simulink model "DvrSimKeybdGD_cs"  (R2016a)
settings: Solver=ode5  SolverMode=SingleTasking  StartTime=0.0  StopTime=inf  FixedStep=1/1000  RelTol=1e-3
PreLoadFcn:
  | mbxruntime.callbacks.PreLoadFcn(bdroot);
PostLoadFcn:
  | mbxruntime.callbacks.PostLoadFcn(bdroot);
InitFcn:
  | mbxruntime.callbacks.InitFcn(bdroot);
StartFcn:
  | mbxruntime.callbacks.StartFcn(bdroot);
StopFcn:
  | mbxruntime.callbacks.StopFcn(bdroot);
model workspace (MAT data in the model file):
  mbox_table : struct (value not decoded)
  model_closed = 0
  sim_status = 0
undefined symbols (not defined in the file or in its folder): BMotor1, BMotor2, BrkDelayTime, DControlB, Delay1, Delay2, DiscIntNeverNeededParam, IControlB, JMotor1, JMotor2, PControlB, PreScanCarSimLoadFcn, ratioGearF, ratioGearR, TorqDelayTime, Tstep
undefined symbols (not defined in the file): SteeringColumn, SteeringWheel, WheelL0, WheelL1, WheelR0, WheelR1
libraries: PreScanSimulinkLibrary x35, simulink_extras x26, simulink x26, MyLib x3, Solver_SF x2, pil_lib x1, PreScanUsefulBlocks x1
(part 12 of 12)

== system DvrSimKeybdGD_cs/Audi_A8_Sedan_1/Trajectories/ElapsedTrack1/MuxState/Substitute 90 & 270 deg (and its plurals)/Angle 0-360 deg limiter ==
  Angle [deg] : Inport
  Gain : Gain  Gain=1/360
  Gain1 : Gain  Gain=360
  Rounding Function : Rounding
  Sum : Sum  Inputs=|-+
  LimAngle [deg] : Outport
  wires:
  Gain/1 -> Rounding Function/1
  Rounding Function/1 -> Gain1/1
  Gain1/1 -> Sum/1
  Angle [deg]/1 -> Gain/1, Sum/2
  Sum/1 -> LimAngle [deg]/1

== system DvrSimKeybdGD_cs/Audi_A8_Sedan_1/Trajectories/Traj2State1/Traj2State2/Traj2MuxState_Ext/demux ==
  traj : Inport
  Demux : Demux  Outputs=18
  x : Outport
  y : Outport  Port=2
  z : Outport  Port=3
  velx : Outport  Port=4
  vely : Outport  Port=5
  velz : Outport  Port=6
  R : Outport  Port=7
  P : Outport  Port=8
  Y : Outport  Port=9
  velR : Outport  Port=10
  velP : Outport  Port=11
  velY : Outport  Port=12
  accx : Outport  Port=13
  accy : Outport  Port=14
  accz : Outport  Port=15
  accR : Outport  Port=16
  accP : Outport  Port=17
  accY : Outport  Port=18
  wires:
  Demux/18 -> accY/1
  Demux/17 -> accP/1
  Demux/16 -> accR/1
  Demux/15 -> accz/1
  Demux/14 -> accy/1
  Demux/13 -> accx/1
  Demux/12 -> velY/1
  Demux/11 -> velP/1
  Demux/10 -> velR/1
  Demux/9 -> velz/1
  Demux/8 -> vely/1
  Demux/7 -> velx/1
  Demux/6 -> Y/1
  Demux/5 -> P/1
  traj/1 -> Demux/1
  Demux/4 -> R/1
  Demux/3 -> z/1
  Demux/2 -> y/1
  Demux/1 -> x/1

== system DvrSimKeybdGD_cs/BMW_X5_SUV_1/Trajectories/ElapsedTrack1/MuxState/Substitute 90 & 270 deg (and its plurals)/Angle 0-360 deg limiter ==
  Angle [deg] : Inport
  Gain : Gain  Gain=1/360
  Gain1 : Gain  Gain=360
  Rounding Function : Rounding
  Sum : Sum  Inputs=|-+
  LimAngle [deg] : Outport
  wires:
  Gain/1 -> Rounding Function/1
  Rounding Function/1 -> Gain1/1
  Gain1/1 -> Sum/1
  Angle [deg]/1 -> Gain/1, Sum/2
  Sum/1 -> LimAngle [deg]/1

== system DvrSimKeybdGD_cs/BMW_X5_SUV_1/Trajectories/Traj2State1/Traj2State2/Traj2MuxState_Ext/demux ==
  traj : Inport
  Demux : Demux  Outputs=18
  x : Outport
  y : Outport  Port=2
  z : Outport  Port=3
  velx : Outport  Port=4
  vely : Outport  Port=5
  velz : Outport  Port=6
  R : Outport  Port=7
  P : Outport  Port=8
  Y : Outport  Port=9
  velR : Outport  Port=10
  velP : Outport  Port=11
  velY : Outport  Port=12
  accx : Outport  Port=13
  accy : Outport  Port=14
  accz : Outport  Port=15
  accR : Outport  Port=16
  accP : Outport  Port=17
  accY : Outport  Port=18
  wires:
  Demux/18 -> accY/1
  Demux/17 -> accP/1
  Demux/16 -> accR/1
  Demux/15 -> accz/1
  Demux/14 -> accy/1
  Demux/13 -> accx/1
  Demux/12 -> velY/1
  Demux/11 -> velP/1
  Demux/10 -> velR/1
  Demux/9 -> velz/1
  Demux/8 -> vely/1
  Demux/7 -> velx/1
  Demux/6 -> Y/1
  Demux/5 -> P/1
  traj/1 -> Demux/1
  Demux/4 -> R/1
  Demux/3 -> z/1
  Demux/2 -> y/1
  Demux/1 -> x/1

== system DvrSimKeybdGD_cs/BMW_Z3_Convertible_1/Trajectories/ElapsedTrack1/MuxState/Substitute 90 & 270 deg (and its plurals)/Angle 0-360 deg limiter ==
  Angle [deg] : Inport
  Gain : Gain  Gain=1/360
  Gain1 : Gain  Gain=360
  Rounding Function : Rounding
  Sum : Sum  Inputs=|-+
  LimAngle [deg] : Outport
  wires:
  Gain/1 -> Rounding Function/1
  Rounding Function/1 -> Gain1/1
  Gain1/1 -> Sum/1
  Angle [deg]/1 -> Gain/1, Sum/2
  Sum/1 -> LimAngle [deg]/1

== system DvrSimKeybdGD_cs/BMW_Z3_Convertible_1/Trajectories/Traj2State1/Traj2State2/Traj2MuxState_Ext/demux ==
  traj : Inport
  Demux : Demux  Outputs=18
  x : Outport
  y : Outport  Port=2
  z : Outport  Port=3
  velx : Outport  Port=4
  vely : Outport  Port=5
  velz : Outport  Port=6
  R : Outport  Port=7
  P : Outport  Port=8
  Y : Outport  Port=9
  velR : Outport  Port=10
  velP : Outport  Port=11
  velY : Outport  Port=12
  accx : Outport  Port=13
  accy : Outport  Port=14
  accz : Outport  Port=15
  accR : Outport  Port=16
  accP : Outport  Port=17
  accY : Outport  Port=18
  wires:
  Demux/18 -> accY/1
  Demux/17 -> accP/1
  Demux/16 -> accR/1
  Demux/15 -> accz/1
  Demux/14 -> accy/1
  Demux/13 -> accx/1
  Demux/12 -> velY/1
  Demux/11 -> velP/1
  Demux/10 -> velR/1
  Demux/9 -> velz/1
  Demux/8 -> vely/1
  Demux/7 -> velx/1
  Demux/6 -> Y/1
  Demux/5 -> P/1
  traj/1 -> Demux/1
  Demux/4 -> R/1
  Demux/3 -> z/1
  Demux/2 -> y/1
  Demux/1 -> x/1

== system DvrSimKeybdGD_cs/Ford_Fiesta_Hatchback_1/Trajectories/ElapsedTrack1/MuxState/Substitute 90 & 270 deg (and its plurals)/Angle 0-360 deg limiter ==
  Angle [deg] : Inport
  Gain : Gain  Gain=1/360
  Gain1 : Gain  Gain=360
  Rounding Function : Rounding
  Sum : Sum  Inputs=|-+
  LimAngle [deg] : Outport
  wires:
  Gain/1 -> Rounding Function/1
  Rounding Function/1 -> Gain1/1
  Gain1/1 -> Sum/1
  Angle [deg]/1 -> Gain/1, Sum/2
  Sum/1 -> LimAngle [deg]/1

== system DvrSimKeybdGD_cs/Ford_Fiesta_Hatchback_1/Trajectories/Traj2State1/Traj2State2/Traj2MuxState_Ext/demux ==
  traj : Inport
  Demux : Demux  Outputs=18
  x : Outport
  y : Outport  Port=2
  z : Outport  Port=3
  velx : Outport  Port=4
  vely : Outport  Port=5
  velz : Outport  Port=6
  R : Outport  Port=7
  P : Outport  Port=8
  Y : Outport  Port=9
  velR : Outport  Port=10
  velP : Outport  Port=11
  velY : Outport  Port=12
  accx : Outport  Port=13
  accy : Outport  Port=14
  accz : Outport  Port=15
  accR : Outport  Port=16
  accP : Outport  Port=17
  accY : Outport  Port=18
  wires:
  Demux/18 -> accY/1
  Demux/17 -> accP/1
  Demux/16 -> accR/1
  Demux/15 -> accz/1
  Demux/14 -> accy/1
  Demux/13 -> accx/1
  Demux/12 -> velY/1
  Demux/11 -> velP/1
  Demux/10 -> velR/1
  Demux/9 -> velz/1
  Demux/8 -> vely/1
  Demux/7 -> velx/1
  Demux/6 -> Y/1
  Demux/5 -> P/1
  traj/1 -> Demux/1
  Demux/4 -> R/1
  Demux/3 -> z/1
  Demux/2 -> y/1
  Demux/1 -> x/1

== system DvrSimKeybdGD_cs/Roewe_550_S_Sedan_1/CarSim_Vehicle/CarSim2PreScan_BUS/Wheel/Convert CarSim to PreScan Wheel Position/Transformation_WheelGlobal2WheelLocal ==
  SprungMass_Pos_Global[x;y;z][m] : Inport
  SprungMass_Angle_Global[x;y;z][deg] : Inport  Port=2
  Wheels_Pos_Global[x;y;z][m] : Inport  Port=3
  D2R : Gain  Gain=pi/180
  Dot Product : DotProduct  InputSameDT=on  OutDataTypeStr=Inherit: Inherit via internal rule
  Dot Product1 : DotProduct  InputSameDT=on  OutDataTypeStr=Inherit: Inherit via internal rule
  Dot Product2 : DotProduct  InputSameDT=on  OutDataTypeStr=Inherit: Inherit via internal rule
  Fcn10 : Fcn  Expr=cos(u(1))*sin(u(2))*sin(u(3))-sin(u(1))*cos(u(3))
  Fcn11 : Fcn  Expr=cos(u(1))*sin(u(2))*cos(u(3))+sin(u(1))*sin(u(3))
  Fcn12 : Fcn  Expr=sin(u(1))*cos(u(2))
  Fcn13 : Fcn  Expr=sin(u(1))*sin(u(2))*sin(u(3))+cos(u(1))*cos(u(3))
  Fcn14 : Fcn  Expr=sin(u(1))*sin(u(2))*cos(u(3))-cos(u(1))*sin(u(3))
  Fcn15 : Fcn  Expr=-sin(u(2))
  Fcn16 : Fcn  Expr=cos(u(2))*sin(u(3))
  Fcn17 : Fcn  Expr=cos(u(2))*cos(u(3))
  Fcn9 : Fcn  Expr=cos(u(1))*cos(u(2))
  Mux : Mux
  Mux1 : Mux  Inputs=9
  Mux3 : Mux  Inputs=3
  PreScan_WheelShiftFL : Subsystem  mask(Translation node configuration){tp=Rear-Left Wheel}
      mask prompts: tp "Type"
      mask init:
      | x_ini_VRML = 2.701790; 
      | y_ini_VRML = 0.665750; 
      | z_ini_VRML = 0.317714;
      mask TypeOptions tp: Front-Left Wheel | Front-Right Wheel | Rear-Left Wheel | Rear-Right Wheel | Left Seat | Right Seat
  PreScan_WheelShiftFR : Subsystem  mask(Translation node configuration){tp=Rear-Right Wheel}
      mask prompts: tp "Type"
      mask init:
      | x_ini_VRML = 2.701790; 
      | y_ini_VRML = -0.665750; 
      | z_ini_VRML = 0.317714;
      mask TypeOptions tp: Front-Left Wheel | Front-Right Wheel | Rear-Left Wheel | Rear-Right Wheel | Left Seat | Right Seat
  PreScan_WheelShiftRL : Subsystem  mask(Translation node configuration){tp=Front-Left Wheel}
      mask prompts: tp "Type"
      mask init:
      | x_ini_VRML = 0.000000; 
      | y_ini_VRML = 0.665750; 
      | z_ini_VRML = 0.317714;
      mask TypeOptions tp: Front-Left Wheel | Front-Right Wheel | Rear-Left Wheel | Rear-Right Wheel | Left Seat | Right Seat
  PreScan_WheelShiftRR : Subsystem  mask(Translation node configuration){tp=Front-Right Wheel}
      mask prompts: tp "Type"
      mask init:
      | x_ini_VRML = 0.000000; 
      | y_ini_VRML = -0.665750; 
      | z_ini_VRML = 0.317714;
      mask TypeOptions tp: Front-Left Wheel | Front-Right Wheel | Rear-Left Wheel | Rear-Right Wheel | Left Seat | Right Seat
  Selector : Selector  InputPortWidth=9  IndexOptions=Index vector (dialog)  Indices=[1 2 3]  OutputSizes=1
  Selector1 : Selector  InputPortWidth=9  IndexOptions=Index vector (dialog)  Indices=[4 5 6]  OutputSizes=1
  Selector2 : Selector  InputPortWidth=9  IndexOptions=Index vector (dialog)  Indices=[7 8 9]  OutputSizes=1
  Subsystem : Subsystem
  Sum{1..4} (4 alike) : Sum  Inputs=-+
  rot_xyz 2 rot_zyx : Selector  InputPortWidth=3  IndexOptions=Index vector (dialog)  Indices=[3 2 1]  OutputSizes=1
  Pos_[FL;FR;RL;RR]_Wheel_CoorSys_V[x;y;z][m] : Outport
  wires:
  PreScan_WheelShiftFL/1(transVisu [m]) -> Mux/1
  PreScan_WheelShiftRL/1(transVisu [m]) -> Mux/3
  PreScan_WheelShiftFR/1(transVisu [m]) -> Mux/2
  D2R/1 -> rot_xyz 2 rot_zyx/1
  Mux/1 -> Pos_[FL;FR;RL;RR]_Wheel_CoorSys_V[x;y;z][m]/1
  PreScan_WheelShiftRR/1(transVisu [m]) -> Mux/4
  [A] -> Sum4/1
  [A] -> Sum2/1
  [A] -> Sum1/1
  Sum4/1 -> PreScan_WheelShiftRR/1(transISO [m])  "WheelRR_Pos_w.r.t._SM_C.S."
  Sum2/1 -> PreScan_WheelShiftRL/1(transISO [m])  "WheelRL_Pos_w.r.t._SM_C.S."
  Sum1/1 -> PreScan_WheelShiftFR/1(transISO [m])  "WheelFR_Pos_w.r.t._SM_C.S."
  Subsystem/4(RR_xyz) -> Sum4/2
  Subsystem/3(RL_xyz) -> Sum2/2
  Subsystem/2(FR_xyz) -> Sum1/2
  Subsystem/1(FL_xyz) -> Sum3/2
  Wheels_Pos_Global[x;y;z][m]/1 -> Subsystem/1(Wheels_Pos_Global[x;y;z][m])
  Sum3/1 -> PreScan_WheelShiftFL/1(transISO [m])  "WheelFL_Pos_w.r.t._SM_C.S."
  SprungMass_Angle_Global[x;y;z][deg]/1 -> D2R/1
  Mux3/1 -> [A], Sum3/1
  rot_xyz 2 rot_zyx/1 -> Fcn16/1, Fcn11/1, Fcn14/1, Fcn17/1, Fcn13/1, Fcn10/1, Fcn15/1, Fcn12/1, Fcn9/1
  Dot Product1/1 -> Mux3/2
  Dot Product2/1 -> Mux3/3
  Selector2/1 -> Subsystem/4(In4), Dot Product2/2
  Selector1/1 -> Subsystem/3(In3), Dot Product1/2
  Dot Product/1 -> Mux3/1
  SprungMass_Pos_Global[x;y;z][m]/1 -> Dot Product/1, Dot Product2/1, Dot Product1/1
  Selector/1 -> Subsystem/2(In2), Dot Product/2
  Mux1/1 -> Selector2/1, Selector1/1, Selector/1  "Inverse RotationMatrix"
  Fcn17/1 -> Mux1/9
  Fcn14/1 -> Mux1/8
  Fcn11/1 -> Mux1/7
  Fcn16/1 -> Mux1/6
  Fcn13/1 -> Mux1/5
  Fcn10/1 -> Mux1/4
  Fcn15/1 -> Mux1/3
  Fcn12/1 -> Mux1/2
  Fcn9/1 -> Mux1/1

== system DvrSimKeybdGD_cs/Roewe_550_S_Sedan_1/CarSim_Vehicle/TyreContact To Road Information/Contact To Road Information/Transformation_PreScan2CarSim/Subsystem ==
  UnitVec_z_CP_CoorSys_PreScan[FL;FR;RL;RR][x;y;z] : Inport
  FirstRow : Inport  Port=2
  SecondRow : Inport  Port=3
  ThirdRow : Inport  Port=4
  Bus Creator{,1..3} (4 alike) : BusCreator  Inputs=3
  Demux1 : Demux  Outputs=[3 3 3 3]
  Dot Product{1..12} (12 alike) : DotProduct  InputSameDT=on  OutDataTypeStr=Inherit: Inherit via internal rule
  UnitVec_z_CP_CoorSys_CarSim[FL][x;y;z] : Outport
  UnitVec_z_CP_CoorSys_CarSim[FR][x;y;z] : Outport  Port=2
  UnitVec_z_CP_CoorSys_CarSim[RL][x;y;z] : Outport  Port=3
  UnitVec_z_CP_CoorSys_CarSim[RR][x;y;z] : Outport  Port=4
  wires:
  [ThirdRow] -> Dot Product12/2
  [ThirdRow] -> Dot Product9/2
  [ThirdRow] -> Dot Product6/2
  [SecondRow] -> Dot Product11/2
  [SecondRow] -> Dot Product8/2
  [SecondRow] -> Dot Product5/2
  FirstRow/1 -> [FirstRow], Dot Product1/2
  [FirstRow] -> Dot Product10/2
  [FirstRow] -> Dot Product7/2
  [FirstRow] -> Dot Product4/2
  Demux1/4 -> Dot Product12/1, Dot Product10/1, Dot Product11/1
  Demux1/3 -> Dot Product9/1, Dot Product7/1, Dot Product8/1
  Demux1/2 -> Dot Product6/1, Dot Product5/1, Dot Product4/1
  Demux1/1 -> Dot Product3/1, Dot Product2/1, Dot Product1/1
  Bus Creator3/1 -> UnitVec_z_CP_CoorSys_CarSim[RR][x;y;z]/1  "UnitVec_z_CP_CoorSys_CarSim[RR][x;y;z]"
  Dot Product11/1 -> Bus Creator3/2  "UnitVec_z_CP_CoorSys_CarSim[RR][y]"
  Dot Product12/1 -> Bus Creator3/3  "UnitVec_z_CP_CoorSys_CarSim[RR][z]"
  Dot Product10/1 -> Bus Creator3/1  "UnitVec_z_CP_CoorSys_CarSim[RR][x]"
  Bus Creator2/1 -> UnitVec_z_CP_CoorSys_CarSim[RL][x;y;z]/1  "UnitVec_z_CP_CoorSys_CarSim[RL][x;y;z]"
  Dot Product8/1 -> Bus Creator2/2  "UnitVec_z_CP_CoorSys_CarSim[RL][y]"
  Dot Product9/1 -> Bus Creator2/3  "UnitVec_z_CP_CoorSys_CarSim[RL][z]"
  Dot Product7/1 -> Bus Creator2/1  "UnitVec_z_CP_CoorSys_CarSim[RL][x]"
  Bus Creator1/1 -> UnitVec_z_CP_CoorSys_CarSim[FR][x;y;z]/1  "UnitVec_z_CP_CoorSys_CarSim[FR][x;y;z]"
  Dot Product5/1 -> Bus Creator1/2  "UnitVec_z_CP_CoorSys_CarSim[FR][y]"
  Dot Product6/1 -> Bus Creator1/3  "UnitVec_z_CP_CoorSys_CarSim[FR][z]"
  Dot Product4/1 -> Bus Creator1/1  "UnitVec_z_CP_CoorSys_CarSim[FR][x]"
  Bus Creator/1 -> UnitVec_z_CP_CoorSys_CarSim[FL][x;y;z]/1  "UnitVec_z_CP_CoorSys_CarSim[FL][x;y;z]"
  Dot Product2/1 -> Bus Creator/2  "UnitVec_z_CP_CoorSys_CarSim[FL][y]"
  Dot Product3/1 -> Bus Creator/3  "UnitVec_z_CP_CoorSys_CarSim[FL][z]"
  Dot Product1/1 -> Bus Creator/1  "UnitVec_z_CP_CoorSys_CarSim[FL][x]"
  UnitVec_z_CP_CoorSys_PreScan[FL;FR;RL;RR][x;y;z]/1 -> Demux1/1
  ThirdRow/1 -> [ThirdRow], Dot Product3/2
  SecondRow/1 -> [SecondRow], Dot Product2/2

== system DvrSimKeybdGD_cs/Roewe_550_S_Sedan_1/PreScan_RayCast_Contact_Sensor/Vehicle Local to World/state2FullState/limit roll/Substitute 90 & 270 deg (and its plurals) ==
  Angle [rad] : Inport
  270 deg detection : simulink/Model Verification/Check  Static Gap  Description=u <= 269.5 || 270.5 <= u  max=270.5  max_included=on  min=269.5  min_included=on  enabled=on  stopWhenAssertionFail=off  export=on  icon=graphic
  90 deg detection : simulink/Model Verification/Check  Static Gap  Description=u <= 89.5 || 90.5 <= u  max=90.5  max_included=on  min=89.5  min_included=on  enabled=on  stopWhenAssertionFail=off  export=on  icon=graphic
  Angle 0-360 deg limiter : Subsystem
  Degrees to Radians : simulink_extras/Transformations/Degrees to Radians
  Radians to Degrees : simulink_extras/Transformations/Radians to Degrees
  Substitution Value : Constant  Value=269.5
  Substitution Value : Constant  Value=89.5
  Switch : Switch  Threshold=0.5
  Switch1 : Switch  Threshold=0.5
  Subst Angle [rad] : Outport
  wires:
  Angle 0-360 deg limiter/1(LimAngle [deg]) -> Switch/1, 90 deg detection/1
  90 deg detection/1 -> Switch/2
  Substitution Value/1 -> Switch/3
  Switch/1 -> 270 deg detection/1, Switch1/1
  270 deg detection/1 -> Switch1/2
  Substitution Value/1 -> Switch1/3
  Switch1/1 -> Degrees to Radians/1
  Radians to Degrees/1 -> Angle 0-360 deg limiter/1(Angle [deg])
  Degrees to Radians/1 -> Subst Angle [rad]/1
  Angle [rad]/1 -> Radians to Degrees/1

== system DvrSimKeybdGD_cs/Roewe_550_S_Sedan_1/PreScan_RayCast_Contact_Sensor1/Vehicle Local to World/state2FullState/limit roll/Substitute 90 & 270 deg (and its plurals) ==
  Angle [rad] : Inport
  270 deg detection : simulink/Model Verification/Check  Static Gap  Description=u <= 269.5 || 270.5 <= u  max=270.5  max_included=on  min=269.5  min_included=on  enabled=on  stopWhenAssertionFail=off  export=on  icon=graphic
  90 deg detection : simulink/Model Verification/Check  Static Gap  Description=u <= 89.5 || 90.5 <= u  max=90.5  max_included=on  min=89.5  min_included=on  enabled=on  stopWhenAssertionFail=off  export=on  icon=graphic
  Angle 0-360 deg limiter : Subsystem
  Degrees to Radians : simulink_extras/Transformations/Degrees to Radians
  Radians to Degrees : simulink_extras/Transformations/Radians to Degrees
  Substitution Value : Constant  Value=269.5
  Substitution Value : Constant  Value=89.5
  Switch : Switch  Threshold=0.5
  Switch1 : Switch  Threshold=0.5
  Subst Angle [rad] : Outport
  wires:
  Angle 0-360 deg limiter/1(LimAngle [deg]) -> Switch/1, 90 deg detection/1
  90 deg detection/1 -> Switch/2
  Substitution Value/1 -> Switch/3
  Switch/1 -> 270 deg detection/1, Switch1/1
  270 deg detection/1 -> Switch1/2
  Substitution Value/1 -> Switch1/3
  Switch1/1 -> Degrees to Radians/1
  Radians to Degrees/1 -> Angle 0-360 deg limiter/1(Angle [deg])
  Degrees to Radians/1 -> Subst Angle [rad]/1
  Angle [rad]/1 -> Radians to Degrees/1

== system DvrSimKeybdGD_cs/Roewe_550_S_Sedan_1/Subsystem/TyreContact To Road Information/Contact To Road Information/Transformation_PreScan2CarSim/Subsystem ==
  UnitVec_z_CP_CoorSys_PreScan[FL;FR;RL;RR][x;y;z] : Inport
  FirstRow : Inport  Port=2
  SecondRow : Inport  Port=3
  ThirdRow : Inport  Port=4
  Bus Creator{,1..3} (4 alike) : BusCreator  Inputs=3
  Demux1 : Demux  Outputs=[3 3 3 3]
  Dot Product{1..12} (12 alike) : DotProduct  InputSameDT=on  OutDataTypeStr=Inherit: Inherit via internal rule
  UnitVec_z_CP_CoorSys_CarSim[FL][x;y;z] : Outport
  UnitVec_z_CP_CoorSys_CarSim[FR][x;y;z] : Outport  Port=2
  UnitVec_z_CP_CoorSys_CarSim[RL][x;y;z] : Outport  Port=3
  UnitVec_z_CP_CoorSys_CarSim[RR][x;y;z] : Outport  Port=4
  wires:
  [ThirdRow] -> Dot Product12/2
  [ThirdRow] -> Dot Product9/2
  [ThirdRow] -> Dot Product6/2
  [SecondRow] -> Dot Product11/2
  [SecondRow] -> Dot Product8/2
  [SecondRow] -> Dot Product5/2
  FirstRow/1 -> [FirstRow], Dot Product1/2
  [FirstRow] -> Dot Product10/2
  [FirstRow] -> Dot Product7/2
  [FirstRow] -> Dot Product4/2
  Demux1/4 -> Dot Product12/1, Dot Product10/1, Dot Product11/1
  Demux1/3 -> Dot Product9/1, Dot Product7/1, Dot Product8/1
  Demux1/2 -> Dot Product6/1, Dot Product5/1, Dot Product4/1
  Demux1/1 -> Dot Product3/1, Dot Product2/1, Dot Product1/1
  Bus Creator3/1 -> UnitVec_z_CP_CoorSys_CarSim[RR][x;y;z]/1  "UnitVec_z_CP_CoorSys_CarSim[RR][x;y;z]"
  Dot Product11/1 -> Bus Creator3/2  "UnitVec_z_CP_CoorSys_CarSim[RR][y]"
  Dot Product12/1 -> Bus Creator3/3  "UnitVec_z_CP_CoorSys_CarSim[RR][z]"
  Dot Product10/1 -> Bus Creator3/1  "UnitVec_z_CP_CoorSys_CarSim[RR][x]"
  Bus Creator2/1 -> UnitVec_z_CP_CoorSys_CarSim[RL][x;y;z]/1  "UnitVec_z_CP_CoorSys_CarSim[RL][x;y;z]"
  Dot Product8/1 -> Bus Creator2/2  "UnitVec_z_CP_CoorSys_CarSim[RL][y]"
  Dot Product9/1 -> Bus Creator2/3  "UnitVec_z_CP_CoorSys_CarSim[RL][z]"
  Dot Product7/1 -> Bus Creator2/1  "UnitVec_z_CP_CoorSys_CarSim[RL][x]"
  Bus Creator1/1 -> UnitVec_z_CP_CoorSys_CarSim[FR][x;y;z]/1  "UnitVec_z_CP_CoorSys_CarSim[FR][x;y;z]"
  Dot Product5/1 -> Bus Creator1/2  "UnitVec_z_CP_CoorSys_CarSim[FR][y]"
  Dot Product6/1 -> Bus Creator1/3  "UnitVec_z_CP_CoorSys_CarSim[FR][z]"
  Dot Product4/1 -> Bus Creator1/1  "UnitVec_z_CP_CoorSys_CarSim[FR][x]"
  Bus Creator/1 -> UnitVec_z_CP_CoorSys_CarSim[FL][x;y;z]/1  "UnitVec_z_CP_CoorSys_CarSim[FL][x;y;z]"
  Dot Product2/1 -> Bus Creator/2  "UnitVec_z_CP_CoorSys_CarSim[FL][y]"
  Dot Product3/1 -> Bus Creator/3  "UnitVec_z_CP_CoorSys_CarSim[FL][z]"
  Dot Product1/1 -> Bus Creator/1  "UnitVec_z_CP_CoorSys_CarSim[FL][x]"
  UnitVec_z_CP_CoorSys_PreScan[FL;FR;RL;RR][x;y;z]/1 -> Demux1/1
  ThirdRow/1 -> [ThirdRow], Dot Product3/2
  SecondRow/1 -> [SecondRow], Dot Product2/2

== system DvrSimKeybdGD_cs/Roewe_550_S_Sedan_1/Subsystem1/CarSim2PreScan_BUS/Wheel/Convert CarSim to PreScan Wheel Position/Transformation_WheelGlobal2WheelLocal ==
  SprungMass_Pos_Global[x;y;z][m] : Inport
  SprungMass_Angle_Global[x;y;z][deg] : Inport  Port=2
  Wheels_Pos_Global[x;y;z][m] : Inport  Port=3
  D2R : Gain  Gain=pi/180
  Dot Product : DotProduct  InputSameDT=on  OutDataTypeStr=Inherit: Inherit via internal rule
  Dot Product1 : DotProduct  InputSameDT=on  OutDataTypeStr=Inherit: Inherit via internal rule
  Dot Product2 : DotProduct  InputSameDT=on  OutDataTypeStr=Inherit: Inherit via internal rule
  Fcn10 : Fcn  Expr=cos(u(1))*sin(u(2))*sin(u(3))-sin(u(1))*cos(u(3))
  Fcn11 : Fcn  Expr=cos(u(1))*sin(u(2))*cos(u(3))+sin(u(1))*sin(u(3))
  Fcn12 : Fcn  Expr=sin(u(1))*cos(u(2))
  Fcn13 : Fcn  Expr=sin(u(1))*sin(u(2))*sin(u(3))+cos(u(1))*cos(u(3))
  Fcn14 : Fcn  Expr=sin(u(1))*sin(u(2))*cos(u(3))-cos(u(1))*sin(u(3))
  Fcn15 : Fcn  Expr=-sin(u(2))
  Fcn16 : Fcn  Expr=cos(u(2))*sin(u(3))
  Fcn17 : Fcn  Expr=cos(u(2))*cos(u(3))
  Fcn9 : Fcn  Expr=cos(u(1))*cos(u(2))
  Mux : Mux
  Mux1 : Mux  Inputs=9
  Mux3 : Mux  Inputs=3
  PreScan_WheelShiftFL : Subsystem  mask(Translation node configuration){tp=Rear-Left Wheel}
      mask prompts: tp "Type"
      mask init:
      | x_ini_VRML = 2.701790; 
      | y_ini_VRML = 0.665750; 
      | z_ini_VRML = 0.317714;
      mask TypeOptions tp: Front-Left Wheel | Front-Right Wheel | Rear-Left Wheel | Rear-Right Wheel | Left Seat | Right Seat
  PreScan_WheelShiftFR : Subsystem  mask(Translation node configuration){tp=Rear-Right Wheel}
      mask prompts: tp "Type"
      mask init:
      | x_ini_VRML = 2.701790; 
      | y_ini_VRML = -0.665750; 
      | z_ini_VRML = 0.317714;
      mask TypeOptions tp: Front-Left Wheel | Front-Right Wheel | Rear-Left Wheel | Rear-Right Wheel | Left Seat | Right Seat
  PreScan_WheelShiftRL : Subsystem  mask(Translation node configuration){tp=Front-Left Wheel}
      mask prompts: tp "Type"
      mask init:
      | x_ini_VRML = 0.000000; 
      | y_ini_VRML = 0.665750; 
      | z_ini_VRML = 0.317714;
      mask TypeOptions tp: Front-Left Wheel | Front-Right Wheel | Rear-Left Wheel | Rear-Right Wheel | Left Seat | Right Seat
  PreScan_WheelShiftRR : Subsystem  mask(Translation node configuration){tp=Front-Right Wheel}
      mask prompts: tp "Type"
      mask init:
      | x_ini_VRML = 0.000000; 
      | y_ini_VRML = -0.665750; 
      | z_ini_VRML = 0.317714;
      mask TypeOptions tp: Front-Left Wheel | Front-Right Wheel | Rear-Left Wheel | Rear-Right Wheel | Left Seat | Right Seat
  Selector : Selector  InputPortWidth=9  IndexOptions=Index vector (dialog)  Indices=[1 2 3]  OutputSizes=1
  Selector1 : Selector  InputPortWidth=9  IndexOptions=Index vector (dialog)  Indices=[4 5 6]  OutputSizes=1
  Selector2 : Selector  InputPortWidth=9  IndexOptions=Index vector (dialog)  Indices=[7 8 9]  OutputSizes=1
  Subsystem : Subsystem
  Sum{1..4} (4 alike) : Sum  Inputs=-+
  rot_xyz 2 rot_zyx : Selector  InputPortWidth=3  IndexOptions=Index vector (dialog)  Indices=[3 2 1]  OutputSizes=1
  Pos_[FL;FR;RL;RR]_Wheel_CoorSys_V[x;y;z][m] : Outport
  wires:
  PreScan_WheelShiftFL/1(transVisu [m]) -> Mux/1
  PreScan_WheelShiftRL/1(transVisu [m]) -> Mux/3
  PreScan_WheelShiftFR/1(transVisu [m]) -> Mux/2
  D2R/1 -> rot_xyz 2 rot_zyx/1
  Mux/1 -> Pos_[FL;FR;RL;RR]_Wheel_CoorSys_V[x;y;z][m]/1
  PreScan_WheelShiftRR/1(transVisu [m]) -> Mux/4
  [A] -> Sum4/1
  [A] -> Sum2/1
  [A] -> Sum1/1
  Sum4/1 -> PreScan_WheelShiftRR/1(transISO [m])  "WheelRR_Pos_w.r.t._SM_C.S."
  Sum2/1 -> PreScan_WheelShiftRL/1(transISO [m])  "WheelRL_Pos_w.r.t._SM_C.S."
  Sum1/1 -> PreScan_WheelShiftFR/1(transISO [m])  "WheelFR_Pos_w.r.t._SM_C.S."
  Subsystem/4(RR_xyz) -> Sum4/2
  Subsystem/3(RL_xyz) -> Sum2/2
  Subsystem/2(FR_xyz) -> Sum1/2
  Subsystem/1(FL_xyz) -> Sum3/2
  Wheels_Pos_Global[x;y;z][m]/1 -> Subsystem/1(Wheels_Pos_Global[x;y;z][m])
  Sum3/1 -> PreScan_WheelShiftFL/1(transISO [m])  "WheelFL_Pos_w.r.t._SM_C.S."
  SprungMass_Angle_Global[x;y;z][deg]/1 -> D2R/1
  Mux3/1 -> [A], Sum3/1
  rot_xyz 2 rot_zyx/1 -> Fcn16/1, Fcn11/1, Fcn14/1, Fcn17/1, Fcn13/1, Fcn10/1, Fcn15/1, Fcn12/1, Fcn9/1
  Dot Product1/1 -> Mux3/2
  Dot Product2/1 -> Mux3/3
  Selector2/1 -> Subsystem/4(In4), Dot Product2/2
  Selector1/1 -> Subsystem/3(In3), Dot Product1/2
  Dot Product/1 -> Mux3/1
  SprungMass_Pos_Global[x;y;z][m]/1 -> Dot Product/1, Dot Product2/1, Dot Product1/1
  Selector/1 -> Subsystem/2(In2), Dot Product/2
  Mux1/1 -> Selector2/1, Selector1/1, Selector/1  "Inverse RotationMatrix"
  Fcn17/1 -> Mux1/9
  Fcn14/1 -> Mux1/8
  Fcn11/1 -> Mux1/7
  Fcn16/1 -> Mux1/6
  Fcn13/1 -> Mux1/5
  Fcn10/1 -> Mux1/4
  Fcn15/1 -> Mux1/3
  Fcn12/1 -> Mux1/2
  Fcn9/1 -> Mux1/1

== system DvrSimKeybdGD_cs/Roewe_550_S_Sedan_1/CarSim_Vehicle/CarSim2PreScan_BUS/Wheel/Convert CarSim to PreScan Wheel Position/Transformation_WheelGlobal2WheelLocal/PreScan_WheelShiftFL ==
  transISO [m] : Inport
  Sum : Sum  Inputs=|+-
  pos_ini_Visu : Subsystem
  transVisu [m] : Outport
  wires:
  Sum/1 -> transVisu [m]/1
  pos_ini_Visu/1(pos_ini_Visu) -> Sum/2
  transISO [m]/1 -> Sum/1

== system DvrSimKeybdGD_cs/Roewe_550_S_Sedan_1/CarSim_Vehicle/CarSim2PreScan_BUS/Wheel/Convert CarSim to PreScan Wheel Position/Transformation_WheelGlobal2WheelLocal/PreScan_WheelShiftFR ==
  transISO [m] : Inport
  Sum : Sum  Inputs=|+-
  pos_ini_Visu : Subsystem
  transVisu [m] : Outport
  wires:
  Sum/1 -> transVisu [m]/1
  pos_ini_Visu/1(pos_ini_Visu) -> Sum/2
  transISO [m]/1 -> Sum/1

== system DvrSimKeybdGD_cs/Roewe_550_S_Sedan_1/CarSim_Vehicle/CarSim2PreScan_BUS/Wheel/Convert CarSim to PreScan Wheel Position/Transformation_WheelGlobal2WheelLocal/PreScan_WheelShiftRL ==
  transISO [m] : Inport
  Sum : Sum  Inputs=|+-
  pos_ini_Visu : Subsystem
  transVisu [m] : Outport
  wires:
  Sum/1 -> transVisu [m]/1
  pos_ini_Visu/1(pos_ini_Visu) -> Sum/2
  transISO [m]/1 -> Sum/1

== system DvrSimKeybdGD_cs/Roewe_550_S_Sedan_1/CarSim_Vehicle/CarSim2PreScan_BUS/Wheel/Convert CarSim to PreScan Wheel Position/Transformation_WheelGlobal2WheelLocal/PreScan_WheelShiftRR ==
  transISO [m] : Inport
  Sum : Sum  Inputs=|+-
  pos_ini_Visu : Subsystem
  transVisu [m] : Outport
  wires:
  Sum/1 -> transVisu [m]/1
  pos_ini_Visu/1(pos_ini_Visu) -> Sum/2
  transISO [m]/1 -> Sum/1

== system DvrSimKeybdGD_cs/Roewe_550_S_Sedan_1/CarSim_Vehicle/CarSim2PreScan_BUS/Wheel/Convert CarSim to PreScan Wheel Position/Transformation_WheelGlobal2WheelLocal/Subsystem ==
  Wheels_Pos_Global[x;y;z][m] : Inport
  In2 : Inport  Port=2
  In3 : Inport  Port=3
  In4 : Inport  Port=4
  Demux1 : Demux  Outputs=[3 3 3 3]
  Dot Product{1..12} (12 alike) : DotProduct  InputSameDT=on  OutDataTypeStr=Inherit: Inherit via internal rule
  Mux{1..4} (4 alike) : Mux  Inputs=3
  FL_xyz : Outport
  FR_xyz : Outport  Port=2
  RL_xyz : Outport  Port=3
  RR_xyz : Outport  Port=4
  wires:
  [ThirdRow] -> Dot Product12/2
  [ThirdRow] -> Dot Product9/2
  [ThirdRow] -> Dot Product6/2
  [SecondRow] -> Dot Product11/2
  [SecondRow] -> Dot Product8/2
  [SecondRow] -> Dot Product5/2
  In2/1 -> [FirstRow], Dot Product1/2
  [FirstRow] -> Dot Product10/2
  [FirstRow] -> Dot Product7/2
  [FirstRow] -> Dot Product4/2
  Demux1/4 -> Dot Product12/1, Dot Product10/1, Dot Product11/1
  Demux1/3 -> Dot Product9/1, Dot Product7/1, Dot Product8/1
  Demux1/2 -> Dot Product6/1, Dot Product5/1, Dot Product4/1
  Demux1/1 -> Dot Product3/1, Dot Product2/1, Dot Product1/1
  Mux4/1 -> RR_xyz/1
  Dot Product11/1 -> Mux4/2
  Dot Product12/1 -> Mux4/3
  Dot Product10/1 -> Mux4/1
  Mux3/1 -> RL_xyz/1
  Dot Product8/1 -> Mux3/2
  Dot Product9/1 -> Mux3/3
  Dot Product7/1 -> Mux3/1
  Mux1/1 -> FR_xyz/1
  Dot Product5/1 -> Mux1/2
  Dot Product6/1 -> Mux1/3
  Dot Product4/1 -> Mux1/1
  Mux2/1 -> FL_xyz/1
  Dot Product2/1 -> Mux2/2
  Dot Product3/1 -> Mux2/3
  Dot Product1/1 -> Mux2/1
  Wheels_Pos_Global[x;y;z][m]/1 -> Demux1/1
  In4/1 -> [ThirdRow], Dot Product3/2
  In3/1 -> [SecondRow], Dot Product2/2

== system DvrSimKeybdGD_cs/Roewe_550_S_Sedan_1/PreScan_RayCast_Contact_Sensor/Vehicle Local to World/state2FullState/limit roll/Substitute 90 & 270 deg (and its plurals)/Angle 0-360 deg limiter ==
  Angle [deg] : Inport
  Gain : Gain  Gain=1/360
  Gain1 : Gain  Gain=360
  Rounding Function : Rounding
  Sum : Sum  Inputs=|-+
  LimAngle [deg] : Outport
  wires:
  Sum/1 -> LimAngle [deg]/1
  Angle [deg]/1 -> Sum/2, Gain/1
  Gain1/1 -> Sum/1
  Rounding Function/1 -> Gain1/1
  Gain/1 -> Rounding Function/1

== system DvrSimKeybdGD_cs/Roewe_550_S_Sedan_1/PreScan_RayCast_Contact_Sensor1/Vehicle Local to World/state2FullState/limit roll/Substitute 90 & 270 deg (and its plurals)/Angle 0-360 deg limiter ==
  Angle [deg] : Inport
  Gain : Gain  Gain=1/360
  Gain1 : Gain  Gain=360
  Rounding Function : Rounding
  Sum : Sum  Inputs=|-+
  LimAngle [deg] : Outport
  wires:
  Sum/1 -> LimAngle [deg]/1
  Angle [deg]/1 -> Sum/2, Gain/1
  Gain1/1 -> Sum/1
  Rounding Function/1 -> Gain1/1
  Gain/1 -> Rounding Function/1

== system DvrSimKeybdGD_cs/Roewe_550_S_Sedan_1/Subsystem1/CarSim2PreScan_BUS/Wheel/Convert CarSim to PreScan Wheel Position/Transformation_WheelGlobal2WheelLocal/PreScan_WheelShiftFL ==
  transISO [m] : Inport
  Sum : Sum  Inputs=|+-
  pos_ini_Visu : Subsystem
  transVisu [m] : Outport
  wires:
  Sum/1 -> transVisu [m]/1
  pos_ini_Visu/1(pos_ini_Visu) -> Sum/2
  transISO [m]/1 -> Sum/1

== system DvrSimKeybdGD_cs/Roewe_550_S_Sedan_1/Subsystem1/CarSim2PreScan_BUS/Wheel/Convert CarSim to PreScan Wheel Position/Transformation_WheelGlobal2WheelLocal/PreScan_WheelShiftFR ==
  transISO [m] : Inport
  Sum : Sum  Inputs=|+-
  pos_ini_Visu : Subsystem
  transVisu [m] : Outport
  wires:
  Sum/1 -> transVisu [m]/1
  pos_ini_Visu/1(pos_ini_Visu) -> Sum/2
  transISO [m]/1 -> Sum/1

== system DvrSimKeybdGD_cs/Roewe_550_S_Sedan_1/Subsystem1/CarSim2PreScan_BUS/Wheel/Convert CarSim to PreScan Wheel Position/Transformation_WheelGlobal2WheelLocal/PreScan_WheelShiftRL ==
  transISO [m] : Inport
  Sum : Sum  Inputs=|+-
  pos_ini_Visu : Subsystem
  transVisu [m] : Outport
  wires:
  Sum/1 -> transVisu [m]/1
  pos_ini_Visu/1(pos_ini_Visu) -> Sum/2
  transISO [m]/1 -> Sum/1

== system DvrSimKeybdGD_cs/Roewe_550_S_Sedan_1/Subsystem1/CarSim2PreScan_BUS/Wheel/Convert CarSim to PreScan Wheel Position/Transformation_WheelGlobal2WheelLocal/PreScan_WheelShiftRR ==
  transISO [m] : Inport
  Sum : Sum  Inputs=|+-
  pos_ini_Visu : Subsystem
  transVisu [m] : Outport
  wires:
  Sum/1 -> transVisu [m]/1
  pos_ini_Visu/1(pos_ini_Visu) -> Sum/2
  transISO [m]/1 -> Sum/1

== system DvrSimKeybdGD_cs/Roewe_550_S_Sedan_1/Subsystem1/CarSim2PreScan_BUS/Wheel/Convert CarSim to PreScan Wheel Position/Transformation_WheelGlobal2WheelLocal/Subsystem ==
  Wheels_Pos_Global[x;y;z][m] : Inport
  In2 : Inport  Port=2
  In3 : Inport  Port=3
  In4 : Inport  Port=4
  Demux1 : Demux  Outputs=[3 3 3 3]
  Dot Product{1..12} (12 alike) : DotProduct  InputSameDT=on  OutDataTypeStr=Inherit: Inherit via internal rule
  Mux{1..4} (4 alike) : Mux  Inputs=3
  FL_xyz : Outport
  FR_xyz : Outport  Port=2
  RL_xyz : Outport  Port=3
  RR_xyz : Outport  Port=4
  wires:
  [ThirdRow] -> Dot Product12/2
  [ThirdRow] -> Dot Product9/2
  [ThirdRow] -> Dot Product6/2
  [SecondRow] -> Dot Product11/2
  [SecondRow] -> Dot Product8/2
  [SecondRow] -> Dot Product5/2
  In2/1 -> [FirstRow], Dot Product1/2
  [FirstRow] -> Dot Product10/2
  [FirstRow] -> Dot Product7/2
  [FirstRow] -> Dot Product4/2
  Demux1/4 -> Dot Product12/1, Dot Product10/1, Dot Product11/1
  Demux1/3 -> Dot Product9/1, Dot Product7/1, Dot Product8/1
  Demux1/2 -> Dot Product6/1, Dot Product5/1, Dot Product4/1
  Demux1/1 -> Dot Product3/1, Dot Product2/1, Dot Product1/1
  Mux4/1 -> RR_xyz/1
  Dot Product11/1 -> Mux4/2
  Dot Product12/1 -> Mux4/3
  Dot Product10/1 -> Mux4/1
  Mux3/1 -> RL_xyz/1
  Dot Product8/1 -> Mux3/2
  Dot Product9/1 -> Mux3/3
  Dot Product7/1 -> Mux3/1
  Mux1/1 -> FR_xyz/1
  Dot Product5/1 -> Mux1/2
  Dot Product6/1 -> Mux1/3
  Dot Product4/1 -> Mux1/1
  Mux2/1 -> FL_xyz/1
  Dot Product2/1 -> Mux2/2
  Dot Product3/1 -> Mux2/3
  Dot Product1/1 -> Mux2/1
  Wheels_Pos_Global[x;y;z][m]/1 -> Demux1/1
  In4/1 -> [ThirdRow], Dot Product3/2
  In3/1 -> [SecondRow], Dot Product2/2

== system DvrSimKeybdGD_cs/Roewe_550_S_Sedan_1/CarSim_Vehicle/CarSim2PreScan_BUS/Wheel/Convert CarSim to PreScan Wheel Position/Transformation_WheelGlobal2WheelLocal/PreScan_WheelShiftFL/pos_ini_Visu ==
  Constant : Constant  Value=x_ini_VRML
  Constant1 : Constant  Value=y_ini_VRML
  Constant2 : Constant  Value=TyreRadius-cogZOffset
  Mux1 : Mux  Inputs=3
  pos_ini_Visu : Outport
  wires:
  Constant2/1 -> Mux1/3
  Constant1/1 -> Mux1/2
  Mux1/1 -> pos_ini_Visu/1
  Constant/1 -> Mux1/1

== system DvrSimKeybdGD_cs/Roewe_550_S_Sedan_1/CarSim_Vehicle/CarSim2PreScan_BUS/Wheel/Convert CarSim to PreScan Wheel Position/Transformation_WheelGlobal2WheelLocal/PreScan_WheelShiftFR/pos_ini_Visu ==
  Constant : Constant  Value=x_ini_VRML
  Constant1 : Constant  Value=y_ini_VRML
  Constant2 : Constant  Value=TyreRadius-cogZOffset
  Mux1 : Mux  Inputs=3
  pos_ini_Visu : Outport
  wires:
  Constant/1 -> Mux1/1
  Mux1/1 -> pos_ini_Visu/1
  Constant1/1 -> Mux1/2
  Constant2/1 -> Mux1/3

== system DvrSimKeybdGD_cs/Roewe_550_S_Sedan_1/CarSim_Vehicle/CarSim2PreScan_BUS/Wheel/Convert CarSim to PreScan Wheel Position/Transformation_WheelGlobal2WheelLocal/PreScan_WheelShiftRL/pos_ini_Visu ==
  Constant : Constant  Value=-x_ini_VRML
  Constant1 : Constant  Value=y_ini_VRML
  Constant2 : Constant  Value=TyreRadius-cogZOffset
  Mux1 : Mux  Inputs=3
  pos_ini_Visu : Outport
  wires:
  Constant/1 -> Mux1/1
  Mux1/1 -> pos_ini_Visu/1
  Constant1/1 -> Mux1/2
  Constant2/1 -> Mux1/3

== system DvrSimKeybdGD_cs/Roewe_550_S_Sedan_1/CarSim_Vehicle/CarSim2PreScan_BUS/Wheel/Convert CarSim to PreScan Wheel Position/Transformation_WheelGlobal2WheelLocal/PreScan_WheelShiftRR/pos_ini_Visu ==
  Constant : Constant  Value=-x_ini_VRML
  Constant1 : Constant  Value=y_ini_VRML
  Constant2 : Constant  Value=TyreRadius-cogZOffset
  Mux1 : Mux  Inputs=3
  pos_ini_Visu : Outport
  wires:
  Constant/1 -> Mux1/1
  Mux1/1 -> pos_ini_Visu/1
  Constant1/1 -> Mux1/2
  Constant2/1 -> Mux1/3

== system DvrSimKeybdGD_cs/Roewe_550_S_Sedan_1/Subsystem1/CarSim2PreScan_BUS/Wheel/Convert CarSim to PreScan Wheel Position/Transformation_WheelGlobal2WheelLocal/PreScan_WheelShiftFL/pos_ini_Visu ==
  Constant : Constant  Value=x_ini_VRML
  Constant1 : Constant  Value=y_ini_VRML
  Constant2 : Constant  Value=TyreRadius-cogZOffset
  Mux1 : Mux  Inputs=3
  pos_ini_Visu : Outport
  wires:
  Constant2/1 -> Mux1/3
  Constant1/1 -> Mux1/2
  Mux1/1 -> pos_ini_Visu/1
  Constant/1 -> Mux1/1

== system DvrSimKeybdGD_cs/Roewe_550_S_Sedan_1/Subsystem1/CarSim2PreScan_BUS/Wheel/Convert CarSim to PreScan Wheel Position/Transformation_WheelGlobal2WheelLocal/PreScan_WheelShiftFR/pos_ini_Visu ==
  Constant : Constant  Value=x_ini_VRML
  Constant1 : Constant  Value=y_ini_VRML
  Constant2 : Constant  Value=TyreRadius-cogZOffset
  Mux1 : Mux  Inputs=3
  pos_ini_Visu : Outport
  wires:
  Constant/1 -> Mux1/1
  Mux1/1 -> pos_ini_Visu/1
  Constant1/1 -> Mux1/2
  Constant2/1 -> Mux1/3

== system DvrSimKeybdGD_cs/Roewe_550_S_Sedan_1/Subsystem1/CarSim2PreScan_BUS/Wheel/Convert CarSim to PreScan Wheel Position/Transformation_WheelGlobal2WheelLocal/PreScan_WheelShiftRL/pos_ini_Visu ==
  Constant : Constant  Value=-x_ini_VRML
  Constant1 : Constant  Value=y_ini_VRML
  Constant2 : Constant  Value=TyreRadius-cogZOffset
  Mux1 : Mux  Inputs=3
  pos_ini_Visu : Outport
  wires:
  Constant/1 -> Mux1/1
  Mux1/1 -> pos_ini_Visu/1
  Constant1/1 -> Mux1/2
  Constant2/1 -> Mux1/3

== system DvrSimKeybdGD_cs/Roewe_550_S_Sedan_1/Subsystem1/CarSim2PreScan_BUS/Wheel/Convert CarSim to PreScan Wheel Position/Transformation_WheelGlobal2WheelLocal/PreScan_WheelShiftRR/pos_ini_Visu ==
  Constant : Constant  Value=-x_ini_VRML
  Constant1 : Constant  Value=y_ini_VRML
  Constant2 : Constant  Value=TyreRadius-cogZOffset
  Mux1 : Mux  Inputs=3
  pos_ini_Visu : Outport
  wires:
  Constant/1 -> Mux1/1
  Mux1/1 -> pos_ini_Visu/1
  Constant1/1 -> Mux1/2
  Constant2/1 -> Mux1/3

== matlab function DvrSimKeybdGD_cs/Roewe_550_S_Sedan_1/CarSim_Vehicle/CarSim2PreScan_ContactAdapter/Embedded MATLAB Function ==
  data: u input; y output
function y = fcn(u)
%#eml

y = norm(u)/3.6;

== matlab function DvrSimKeybdGD_cs/Roewe_550_S_Sedan_1/CarSim I//O/LaneMarker/MATLAB Function ==
  data: Lane3_X input; Lane3_Y input; Lane1_X input; Lane1_Y input; Lane2_X input; Lane2_Y input; Lane1 output; Lane2 output; Lane3 output; Lane4_X input; Lane4_Y input; Lane4 output
function [Lane1,Lane2,Lane3,Lane4] = fcn(Lane3_X,Lane3_Y,Lane1_X,Lane1_Y,Lane2_X,Lane2_Y,Lane4_X,Lane4_Y)
%#codegen

p1 = polyfit(Lane1_X,Lane1_Y,3);
p2 = polyfit(Lane2_X,Lane2_Y,3);
p3 = polyfit(Lane3_X,Lane3_Y,3);
p4 = polyfit(Lane4_X,Lane4_Y,3);

Lane1PosC0_m = single(p1(4));
Lane1HeadAngC1_Rad = single(p1(3));
Lane1LaneCurvC2_1pm = single(p1(2));
Lane1CurvDrivC3_1pms = single(p1(1));

Lane2PosC0_m = single(p2(4));
Lane2HeadAngC1_Rad = single(p2(3));
Lane2LaneCurvC2_1pm = single(p2(2));
Lane2CurvDrivC3_1pms = single(p2(1));

Lane3PosC0_m = single(p3(4));
Lane3HeadAngC1_Rad = single(p3(3));
Lane3LaneCurvC2_1pm = single(p3(2));
Lane3CurvDrivC3_1pms = single(p3(1));

Lane4PosC0_m = single(p4(4));
Lane4HeadAngC1_Rad = single(p4(3));
Lane4LaneCurvC2_1pm = single(p4(2));
Lane4CurvDrivC3_1pms = single(p4(1));
% set lane1 and lane3 x to be negtive
Lane1=-1*[Lane1PosC0_m Lane1HeadAngC1_Rad Lane1LaneCurvC2_1pm Lane1CurvDrivC3_1pms];
Lane2=-1*[Lane2PosC0_m Lane2HeadAngC1_Rad Lane2LaneCurvC2_1pm Lane2CurvDrivC3_1pms];
Lane3=-1*[Lane3PosC0_m Lane3HeadAngC1_Rad Lane3LaneCurvC2_1pm Lane3CurvDrivC3_1pms];
Lane4=-1*[Lane4PosC0_m Lane4HeadAngC1_Rad Lane4LaneCurvC2_1pm Lane4CurvDrivC3_1pms];
end

== matlab function DvrSimKeybdGD_cs/Roewe_550_S_Sedan_1/Subsystem1/CarSim2PreScan_ContactAdapter/Embedded MATLAB Function ==
  data: u input; y output
function y = fcn(u)
%#eml

y = norm(u)/3.6;
